simulink model "platoon_NRMPC"  (R2024b)
settings: Solver=FixedStepAuto  StartTime=0.0  StopTime=240  FixedStep=d_t  RelTol=1e-3
values from neighbouring files (symbols this model uses):
  A_i = [0 1;0 0]    [design_script.m]    (also in platoon_implementation_variables.mat = [0  1; 0  0])
  act_est = cell(1,N)    [design_script.m]    (also in platoon_implementation_variables.mat = )
  amp_n_u_f = 2e-2    (= 0.02)    [design_script.m]    (also in platoon_implementation_variables.mat)
  amp_n_u_s1 = 1e-2    (= 0.01)    [design_script.m]    (also in platoon_implementation_variables.mat)
  amp_n_u_s2 = 1e-2    (= 0.01)    [design_script.m]    (also in platoon_implementation_variables.mat)
  amp_n_x = 1e-2    (= 0.01)    [design_script.m]    (also in platoon_implementation_variables.mat)
  B_i = [0;1]    [design_script.m]    (also in platoon_implementation_variables.mat = [0 1])
  C = [1 0]    [design_script.m]    (also in platoon_implementation_variables.mat)
  car_len_prev = [0 5*ones(1,N-1)]    [design_script.m]    (also in platoon_implementation_variables.mat = [0 5 5 5 5 5 5 5 5 5])
  Ch = [1 h]    [design_script.m]    (also in platoon_implementation_variables.mat = [1 5])
  d_t = 0.1    [design_script.m]    (also in platoon_implementation_variables.mat)
  G_act_c = cell(1,N)    [design_script.m]    (also in platoon_implementation_variables.mat = )
  K_D_implem =     [NRF_implem.mat]    (also in platoon_implementation_variables.mat)
  m = dims(3)    [car_MPC_follower.m]    (also in car_MPC_leader.m = dims(2); platoon_implementation_variables.mat = 1)
  n = dims(2)    [car_MPC_follower.m]    (also in car_MPC_leader.m = dims(1); platoon_implementation_variables.mat = 3)
  n_w = zeros(1,N)    [design_script.m]    (also in platoon_implementation_variables.mat = [1 1 1 1 1 1 1 1 1 1])
  pos_ref = h*10    (= 50)    [design_script.m]    (also in platoon_implementation_variables.mat)
  U_lims = 10 * ones(1,N)    [design_script.m]    (also in platoon_implementation_variables.mat = [10 10 10 10 10 10 10 10 10 10])
  x0_c = [9.38914167955 12.3528095305 0 -60.4298352947 12.5503912552 0 -103.066925889 9.67248980493 0 -164.188527826 9.84551868802 0 ... (30 elements, 3x10)]    [init_scatter.mat]    (also in platoon_implementation_variables.mat)
undefined symbols (not defined in the file or in its folder): car_MPC_follower, car_MPC_leader, DiscIntNeverNeededParam
settings Model: Creator=Andrei

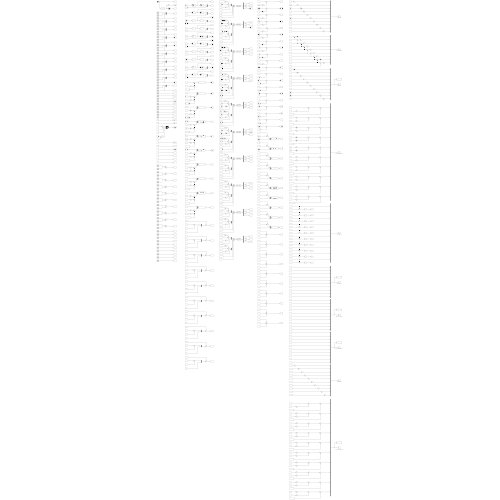
[thumbnail: Simulink's stored preview of the top-level diagram]
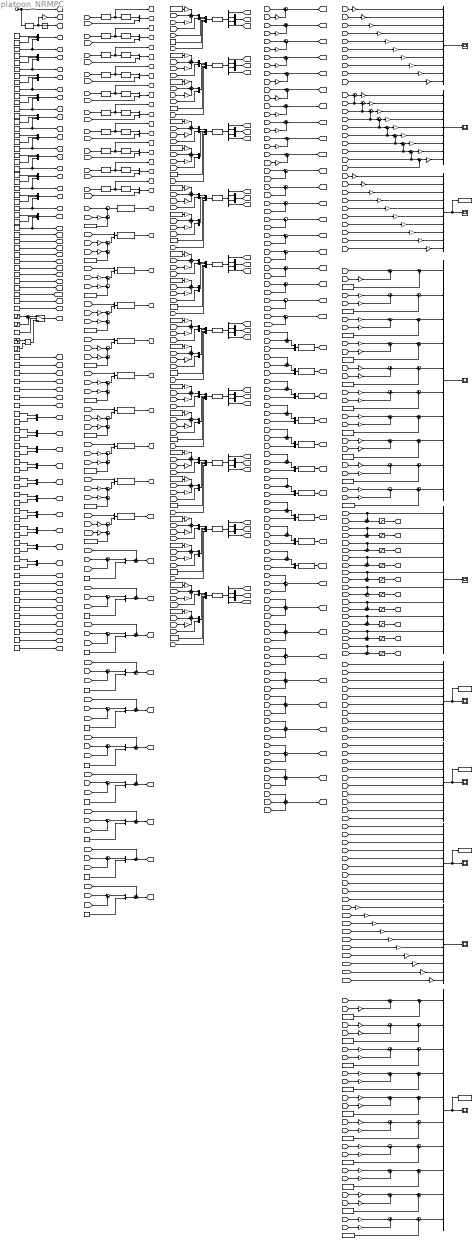
== system platoon_NRMPC ==
  " " : MATLABFcn  MATLABFcn=car_MPC_leader(u(1:n+n_w(1)),u(n+n_w(1)+1),u(n+n_w(1)+2:n+n_w(1)+3),u(n+n_w(1)+4))  OutputDimensions=n+m  SampleTime=d_t
  "  " : MATLABFcn  MATLABFcn=car_MPC_follower(u(1:n+n_w(2)),u(n+n_w(2)+1:2*n+n_w(1)+n_w(2)),u(2*n+n_w(1)+n_w(2)+1:2*n+n_w(1)+n_w(2)+3),u(2*n+n_w(1)+n_w(2)+4))  OutputDimensions=n+m  SampleTime=d_t
  "   " : MATLABFcn  MATLABFcn=car_MPC_follower(u(1:n+n_w(3)),u(n+n_w(3)+1:2*n+n_w(2)+n_w(3)),u(2*n+n_w(2)+n_w(3)+1:2*n+n_w(2)+n_w(3)+3),u(2*n+n_w(2)+n_w(3)+4))  OutputDimensions=n+m  SampleTime=d_t
  "    " : MATLABFcn  MATLABFcn=car_MPC_follower(u(1:n+n_w(4)),u(n+n_w(4)+1:2*n+n_w(3)+n_w(4)),u(2*n+n_w(3)+n_w(4)+1:2*n+n_w(3)+n_w(4)+3),u(2*n+n_w(3)+n_w(4)+4))  OutputDimensions=n+m  SampleTime=d_t
  "     " : MATLABFcn  MATLABFcn=car_MPC_follower(u(1:n+n_w(5)),u(n+n_w(5)+1:2*n+n_w(4)+n_w(5)),u(2*n+n_w(4)+n_w(5)+1:2*n+n_w(4)+n_w(5)+3),u(2*n+n_w(4)+n_w(5)+4))  OutputDimensions=n+m  SampleTime=d_t
  "      " : MATLABFcn  MATLABFcn=car_MPC_follower(u(1:n+n_w(6)),u(n+n_w(6)+1:2*n+n_w(5)+n_w(6)),u(2*n+n_w(5)+n_w(6)+1:2*n+n_w(5)+n_w(6)+3),u(2*n+n_w(5)+n_w(6)+4))  OutputDimensions=n+m  SampleTime=d_t
  "       " : MATLABFcn  MATLABFcn=car_MPC_follower(u(1:n+n_w(7)),u(n+n_w(7)+1:2*n+n_w(6)+n_w(7)),u(2*n+n_w(6)+n_w(7)+1:2*n+n_w(6)+n_w(7)+3),u(2*n+n_w(6)+n_w(7)+4))  OutputDimensions=n+m  SampleTime=d_t
  "        " : MATLABFcn  MATLABFcn=car_MPC_follower(u(1:n+n_w(8)),u(n+n_w(8)+1:2*n+n_w(7)+n_w(8)),u(2*n+n_w(7)+n_w(8)+1:2*n+n_w(7)+n_w(8)+3),u(2*n+n_w(7)+n_w(8)+4))  OutputDimensions=n+m  SampleTime=d_t
  "         " : MATLABFcn  MATLABFcn=car_MPC_follower(u(1:n+n_w(9)),u(n+n_w(9)+1:2*n+n_w(8)+n_w(9)),u(2*n+n_w(8)+n_w(9)+1:2*n+n_w(8)+n_w(9)+3),u(2*n+n_w(8)+n_w(9)+4))  OutputDimensions=n+m  SampleTime=d_t
  "          " : MATLABFcn  MATLABFcn=car_MPC_follower(u(1:n+n_w(10)),u(n+n_w(10)+1:2*n+n_w(9)+n_w(10)),u(2*n+n_w(9)+n_w(10)+1:2*n+n_w(9)+n_w(10)+3),u(2*n+n_w(9)+n_w(10)+4))  OutputDimensions=n+m  SampleTime=d_t
  Clock1 : Clock
  Constant1 : Constant
  Constant{5..6,8..10,18,22..25,51..59} (19 alike) : Constant  Value=0  SampleTime=d_t
  Constant{11,33,37,64,74} (5 alike) : Constant  Value=car_len_prev(5)  SampleTime=d_t
  Constant{12,36,40,65,75} (5 alike) : Constant  Value=car_len_prev(6)  SampleTime=d_t
  Constant{13,39,43,66,76} (5 alike) : Constant  Value=car_len_prev(7)  SampleTime=d_t
  Constant{14,42,46,67,77} (5 alike) : Constant  Value=car_len_prev(8)  SampleTime=d_t
  Constant{15,45,49,68,78} (5 alike) : Constant  Value=car_len_prev(9)  SampleTime=d_t
  Constant{16,48,69,79} (4 alike) : Constant  Value=car_len_prev(10)  SampleTime=d_t
  Constant{2,17,20,60,70} (5 alike) : Constant  Value=car_len_prev(1)  SampleTime=d_t
  Constant{4,19,28,61,71} (5 alike) : Constant  Value=car_len_prev(2)  SampleTime=d_t
  Constant21 : Constant  Value=[n; m]  SampleTime=d_t
  Constant26 : Constant  Value=[2; n; m]  SampleTime=d_t
  Constant{3,27,31,62,72} (5 alike) : Constant  Value=car_len_prev(3)  SampleTime=d_t
  Constant29 : Constant  Value=[3; n; m]  SampleTime=d_t
  Constant{7,30,34,63,73} (5 alike) : Constant  Value=car_len_prev(4)  SampleTime=d_t
  Constant32 : Constant  Value=[4; n; m]  SampleTime=d_t
  Constant35 : Constant  Value=[5; n; m]  SampleTime=d_t
  Constant38 : Constant  Value=[6; n; m]  SampleTime=d_t
  Constant41 : Constant  Value=[7; n; m]  SampleTime=d_t
  Constant44 : Constant  Value=[8; n; m]  SampleTime=d_t
  Constant47 : Constant  Value=[9; n; m]  SampleTime=d_t
  Constant50 : Constant  Value=[10; n; m]  SampleTime=d_t
  Demux{,1..9} (10 alike) : Demux
  Discrete State-Space : DiscreteStateSpace  A=K_D_implem{1}.a  B=K_D_implem{1}.b  C=K_D_implem{1}.c  D=K_D_implem{1}.d  SampleTime=d_t
  Discrete State-Space1 : DiscreteStateSpace  A=K_D_implem{2}.a  B=K_D_implem{2}.b  C=K_D_implem{2}.c  D=K_D_implem{2}.d  SampleTime=d_t
  Discrete State-Space10 : DiscreteStateSpace  A=act_est{1}.a  B=act_est{1}.b  C=act_est{1}.c  D=act_est{1}.d  SampleTime=d_t
  Discrete State-Space11 : DiscreteStateSpace  A=act_est{2}.a  B=act_est{2}.b  C=act_est{2}.c  D=act_est{2}.d  SampleTime=d_t
  Discrete State-Space12 : DiscreteStateSpace  A=act_est{3}.a  B=act_est{3}.b  C=act_est{3}.c  D=act_est{3}.d  SampleTime=d_t
  Discrete State-Space13 : DiscreteStateSpace  A=act_est{4}.a  B=act_est{4}.b  C=act_est{4}.c  D=act_est{4}.d  SampleTime=d_t
  Discrete State-Space14 : DiscreteStateSpace  A=act_est{5}.a  B=act_est{5}.b  C=act_est{5}.c  D=act_est{5}.d  SampleTime=d_t
  Discrete State-Space15 : DiscreteStateSpace  A=act_est{6}.a  B=act_est{6}.b  C=act_est{6}.c  D=act_est{6}.d  SampleTime=d_t
  Discrete State-Space16 : DiscreteStateSpace  A=act_est{7}.a  B=act_est{7}.b  C=act_est{7}.c  D=act_est{7}.d  SampleTime=d_t
  Discrete State-Space17 : DiscreteStateSpace  A=act_est{8}.a  B=act_est{8}.b  C=act_est{8}.c  D=act_est{8}.d  SampleTime=d_t
  Discrete State-Space18 : DiscreteStateSpace  A=act_est{9}.a  B=act_est{9}.b  C=act_est{9}.c  D=act_est{9}.d  SampleTime=d_t
  Discrete State-Space19 : DiscreteStateSpace  A=act_est{10}.a  B=act_est{10}.b  C=act_est{10}.c  D=act_est{10}.d  SampleTime=d_t
  Discrete State-Space2 : DiscreteStateSpace  A=K_D_implem{3}.a  B=K_D_implem{3}.b  C=K_D_implem{3}.c  D=K_D_implem{3}.d  SampleTime=d_t
  Discrete State-Space3 : DiscreteStateSpace  A=K_D_implem{4}.a  B=K_D_implem{4}.b  C=K_D_implem{4}.c  D=K_D_implem{4}.d  SampleTime=d_t
  Discrete State-Space4 : DiscreteStateSpace  A=K_D_implem{5}.a  B=K_D_implem{5}.b  C=K_D_implem{5}.c  D=K_D_implem{5}.d  SampleTime=d_t
  Discrete State-Space5 : DiscreteStateSpace  A=K_D_implem{6}.a  B=K_D_implem{6}.b  C=K_D_implem{6}.c  D=K_D_implem{6}.d  SampleTime=d_t
  Discrete State-Space6 : DiscreteStateSpace  A=K_D_implem{7}.a  B=K_D_implem{7}.b  C=K_D_implem{7}.c  D=K_D_implem{7}.d  SampleTime=d_t
  Discrete State-Space7 : DiscreteStateSpace  A=K_D_implem{8}.a  B=K_D_implem{8}.b  C=K_D_implem{8}.c  D=K_D_implem{8}.d  SampleTime=d_t
  Discrete State-Space8 : DiscreteStateSpace  A=K_D_implem{9}.a  B=K_D_implem{9}.b  C=K_D_implem{9}.c  D=K_D_implem{9}.d  SampleTime=d_t
  Discrete State-Space9 : DiscreteStateSpace  A=K_D_implem{10}.a  B=K_D_implem{10}.b  C=K_D_implem{10}.c  D=K_D_implem{10}.d  SampleTime=d_t
  Discrete-Time Integrator1 : DiscreteIntegrator  InitialCondition=pos_ref  SampleTime=d_t  ICPrevOutput=DiscIntNeverNeededParam  ICPrevScaledInput=DiscIntNeverNeededParam
  Fcn : Fcn  Expr=spd_ref*(u(1)>=0)+(3-spd_ref)*(u(1)>=40)+30*(u(1)>=120)-30*(u(1)>=130)
  Gain{1,3,29,56,58,60,62,64,66,68,139,142..143,145,147,149..150,152,154,157} (20 alike) : Gain  Gain=[Ch 0]  Multiplication=Matrix(K*u)
  Gain{2,4,6..16,18..28,38..39,42..55,57,59,61,63,65,67,71,141,144,146,148,151,153,155..156,158} (56 alike) : Gain  Gain=[C 0]  Multiplication=Matrix(K*u)
  Gain{69,76,78,80,82,84,86,88,90,92,94,96,98,100,102,104,106} (17 alike) : Gain  Gain=blkdiag(1,0,0)  Multiplication=Matrix(K*u)
  Gain{5,70,73..75,77,79,81,83,85,87,89,91,93,95,97,99,101,103,105,107} (21 alike) : Gain  Gain=[1;0;0]  Multiplication=Matrix(K*u)
  Gain108 : Gain  Gain=5  Multiplication=Matrix(K*u)
  Gain109 : Gain  Gain=6  Multiplication=Matrix(K*u)
  Gain110 : Gain  Gain=7  Multiplication=Matrix(K*u)
  Gain{111..120} (10 alike) : Gain  Gain=[0 1 0]  Multiplication=Matrix(K*u)
  Gain121 : Gain  Gain=8  Multiplication=Matrix(K*u)
  Gain122 : Gain  Gain=9  Multiplication=Matrix(K*u)
  Gain123 : Gain  Gain=10  Multiplication=Matrix(K*u)
  Gain124 : Gain  Multiplication=Matrix(K*u)
  Gain125 : Gain  Gain=2  Multiplication=Matrix(K*u)
  Gain126 : Gain  Gain=3  Multiplication=Matrix(K*u)
  Gain127 : Gain  Gain=4  Multiplication=Matrix(K*u)
  Gain17 : Gain  Gain=d_t
  Gain{30..37,40..41} (10 alike) : Gain  Gain=diag([1 1 0])  Multiplication=Matrix(K*u)
  MPC commands to NRF : Scope
  MPC commands to platoon : Scope
  MPC infeasibility : Scope
  Mux{,7..11,22..23,25,27} (10 alike) : Mux  Inputs=3
  Mux{1..6,15..19,21,24,26,28..46,48,50..52,54,56..57,59..61,63..65,67..69,71..73,75..77,79..81,83,85..103} (78 alike) : Mux  Inputs=2
  Mux{13..14,20,55,84,104..107} (9 alike) : Mux  Inputs=10
  Mux12 : Mux  Inputs=9
  Mux{47,49,53,58,62,66,70,74,78,82} (10 alike) : Mux
  NRF commands : Scope
  Product : Product
  Saturation : Saturate  UpperLimit=U_lims(1)  LowerLimit=-U_lims(1)
  Saturation1 : Saturate  UpperLimit=U_lims(2)  LowerLimit=-U_lims(2)
  Saturation2 : Saturate  UpperLimit=U_lims(3)  LowerLimit=-U_lims(3)
  Saturation3 : Saturate  UpperLimit=U_lims(4)  LowerLimit=-U_lims(4)
  Saturation4 : Saturate  UpperLimit=U_lims(5)  LowerLimit=-U_lims(5)
  Saturation5 : Saturate  UpperLimit=U_lims(6)  LowerLimit=-U_lims(6)
  Saturation6 : Saturate  UpperLimit=U_lims(7)  LowerLimit=-U_lims(7)
  Saturation7 : Saturate  UpperLimit=U_lims(8)  LowerLimit=-U_lims(8)
  Saturation8 : Saturate  UpperLimit=U_lims(9)  LowerLimit=-U_lims(9)
  Saturation9 : Saturate  UpperLimit=U_lims(10)  LowerLimit=-U_lims(10)
  Sine Wave : Sin  Amplitude=0.4*U_lims(3)  Frequency=0.2  Phase=pi  SampleTime=d_t
  State-Space : StateSpace  A=A_i  B=B_i  C=eye(2)  D=zeros(2,1)  InitialCondition=x0_c(1:2,1)
  State-Space1 : StateSpace  A=G_act_c{1}.a  B=G_act_c{1}.b  C=G_act_c{1}.c  D=G_act_c{1}.d  InitialCondition=x0_c(3,1)
  State-Space10 : StateSpace  A=A_i  B=B_i  C=eye(2)  D=zeros(2,1)  InitialCondition=x0_c(1:2,6)
  State-Space11 : StateSpace  A=G_act_c{6}.a  B=G_act_c{6}.b  C=G_act_c{6}.c  D=G_act_c{6}.d  InitialCondition=x0_c(3,6)
  State-Space12 : StateSpace  A=A_i  B=B_i  C=eye(2)  D=zeros(2,1)  InitialCondition=x0_c(1:2,10)
  State-Space13 : StateSpace  A=G_act_c{10}.a  B=G_act_c{10}.b  C=G_act_c{10}.c  D=G_act_c{10}.d  InitialCondition=x0_c(3,10)
  State-Space14 : StateSpace  A=A_i  B=B_i  C=eye(2)  D=zeros(2,1)  InitialCondition=x0_c(1:2,7)
  State-Space15 : StateSpace  A=G_act_c{7}.a  B=G_act_c{7}.b  C=G_act_c{7}.c  D=G_act_c{7}.d  InitialCondition=x0_c(3,7)
  State-Space16 : StateSpace  A=A_i  B=B_i  C=eye(2)  D=zeros(2,1)  InitialCondition=x0_c(1:2,8)
  State-Space17 : StateSpace  A=G_act_c{8}.a  B=G_act_c{8}.b  C=G_act_c{8}.c  D=G_act_c{8}.d  InitialCondition=x0_c(3,8)
  State-Space18 : StateSpace  A=A_i  B=B_i  C=eye(2)  D=zeros(2,1)  InitialCondition=x0_c(1:2,9)
  State-Space19 : StateSpace  A=G_act_c{9}.a  B=G_act_c{9}.b  C=G_act_c{9}.c  D=G_act_c{9}.d  InitialCondition=x0_c(3,9)
  State-Space2 : StateSpace  A=A_i  B=B_i  C=eye(2)  D=zeros(2,1)  InitialCondition=x0_c(1:2,2)
  State-Space3 : StateSpace  A=G_act_c{2}.a  B=G_act_c{2}.b  C=G_act_c{2}.c  D=G_act_c{2}.d  InitialCondition=x0_c(3,2)
  State-Space4 : StateSpace  A=A_i  B=B_i  C=eye(2)  D=zeros(2,1)  InitialCondition=x0_c(1:2,3)
  State-Space5 : StateSpace  A=G_act_c{3}.a  B=G_act_c{3}.b  C=G_act_c{3}.c  D=G_act_c{3}.d  InitialCondition=x0_c(3,3)
  State-Space6 : StateSpace  A=A_i  B=B_i  C=eye(2)  D=zeros(2,1)  InitialCondition=x0_c(1:2,4)
  State-Space7 : StateSpace  A=G_act_c{4}.a  B=G_act_c{4}.b  C=G_act_c{4}.c  D=G_act_c{4}.d  InitialCondition=x0_c(3,4)
  State-Space8 : StateSpace  A=A_i  B=B_i  C=eye(2)  D=zeros(2,1)  InitialCondition=x0_c(1:2,5)
  State-Space9 : StateSpace  A=G_act_c{5}.a  B=G_act_c{5}.b  C=G_act_c{5}.c  D=G_act_c{5}.d  InitialCondition=x0_c(3,5)
  Step : Step  Time=40  After=-2*U_lims(3)  SampleTime=d_t
  Step1 : Step  Time=40  After=2*U_lims(3)  SampleTime=d_t
  Step2 : Step  Time=40  SampleTime=d_t
  Sum{,1..2,4..5,8,11,13..14,22,28,30,32,34,36,38,40..44,46,48,53..54,99,109,111,113,115,117,119,121,123,125,127,129,132..133,135,138,140..141,144..145,147,150..152,155..156} (51 alike) : Sum  Inputs=|++
  Sum{3,7,10,52,55,130..131,134,136..137,139,142..143,146,148..149,153..154,157..158} (20 alike) : Sum  Inputs=|-+
  Sum{81,100..108} (10 alike) : Sum  Inputs=+++
  Sum{29,31,33,35,37,39,45,47,49..51,60..78,110,112,114,116,118,120,122,124,126,128} (40 alike) : Sum  Inputs=++|
  Sum{6,9,12,15..21,23..27,56..59} (19 alike) : Sum  Inputs=|+-
  Sum{79..80,82..98} (19 alike) : Sum  Inputs=++-
  Switch : Switch  Criteria=u2 > Threshold  SaturateOnIntegerOverflow=off  InputSameDT=off
  To Workspace : ToWorkspace  VariableName=y  SaveFormat=Timeseries  SampleTime=d_t
  To Workspace1 : ToWorkspace  VariableName=u_s2  SaveFormat=Timeseries  SampleTime=d_t
  To Workspace2 : ToWorkspace  VariableName=u_s1  SaveFormat=Timeseries  SampleTime=d_t
  To Workspace3 : ToWorkspace  VariableName=u_f  SaveFormat=Timeseries  SampleTime=d_t
  To Workspace4 : ToWorkspace  VariableName=v  SaveFormat=Timeseries  SampleTime=d_t
  Uniform Random Number{,1..17,28..39} (30 alike) : UniformRandomNumber  Minimum=-amp_n_x  Maximum=amp_n_x  Seed=randi(1e3)  SampleTime=d_t
  Uniform Random Number{18..27} (10 alike) : UniformRandomNumber  Minimum=-amp_n_u_f  Maximum=amp_n_u_f  Seed=randi(1e3)  SampleTime=d_t
  Uniform Random Number{40..59} (20 alike) : UniformRandomNumber  Minimum=-amp_n_u_s1  Maximum=amp_n_u_s1  Seed=randi(1e3)  SampleTime=d_t
  Uniform Random Number{60..69} (10 alike) : UniformRandomNumber  Minimum=-amp_n_u_s2  Maximum=amp_n_u_s2  Seed=randi(1e3)  SampleTime=d_t
  headway_based_distances : Scope
  intervehicle_distance : Scope
  length_based_interdistances : Scope
  total_commands : Scope
  vehicle position : Scope
  vehicle speed : Scope
  wires:
  Mux12/1 -> intervehicle_distance/1
  Sum29/1 -> Saturation/1
  Sum31/1 -> Saturation1/1
  Sum35/1 -> Saturation3/1
  Sum39/1 -> Saturation5/1
  Sum37/1 -> Saturation4/1
  [d_1] -> Sum29/2
  [d_2] -> Sum31/2
  [d_3] -> Sum33/2
  [d_4] -> Sum35/2
  [d_5] -> Sum37/2
  [d_6] -> Sum39/2
  [x_6] -> Gain11/1
  [x_1] -> Gain6/1
  [x_5] -> Gain10/1
  [x_4] -> Gain9/1
  [x_3] -> Gain8/1
  [x_2] -> Gain7/1
  Mux14/1 -> vehicle position/1
  Gain6/1 -> Mux14/1
  Gain7/1 -> Mux14/2
  Gain8/1 -> Mux14/3
  Gain9/1 -> Mux14/4
  Gain10/1 -> Mux14/5
  Gain11/1 -> Mux14/6
  Sum33/1 -> Saturation2/1
  Uniform Random Number21/1 -> [n_u_f_4]
  Uniform Random Number19/1 -> [n_u_f_2]
  Constant8/1 -> [d_4]
  Constant9/1 -> [d_5]
  Constant6/1 -> [d_2]
  Constant5/1 -> [d_1]
  Uniform Random Number22/1 -> [n_u_f_5]
  Sum/1 -> Switch/1
  Uniform Random Number18/1 -> [n_u_f_1]
  Uniform Random Number23/1 -> [n_u_f_6]
  Step/1 -> Sum/1
  Constant10/1 -> [d_6]
  Step1/1 -> Sum/2
  Uniform Random Number20/1 -> [n_u_f_3]
  Saturation/1 -> [u_1]
  Saturation1/1 -> [u_2]
  Saturation2/1 -> [u_3]
  Saturation3/1 -> [u_4]
  Saturation4/1 -> [u_5]
  Saturation5/1 -> [u_6]
  Sum14/1 -> [x_n_a_6]
  [x_2] -> Sum1/1
  Sum4/1 -> [x_n_a_1]
  [x_4] -> Sum8/1
  [n_x_1] -> Gain31/1
  [n_x_3] -> Gain32/1
  [x_6] -> Sum14/1
  [x_5] -> Sum11/1
  Sum8/1 -> [x_n_a_4]
  Gain31/1 -> Sum4/2
  Sum11/1 -> [x_n_a_5]
  Gain40/1 -> Sum11/2
  Gain41/1 -> Sum14/2
  Gain33/1 -> Sum8/2
  Gain30/1 -> Sum1/2
  [x_1] -> Sum4/1
  Gain32/1 -> Sum5/2
  [x_3] -> Sum5/1
  Sum5/1 -> [x_n_a_3]
  Sum1/1 -> [x_n_a_2]
  [n_x_2] -> Gain30/1
  [n_x_5] -> Gain40/1
  [n_x_4] -> Gain33/1
  [n_x_6] -> Gain41/1
  Mux24/1 -> [x_2]
  Mux30/1 -> [x_5]
  [u_5] -> State-Space9/1
  State-Space8/1 -> Mux30/1
  State-Space11/1 -> [a_6], State-Space10/1
  State-Space3/1 -> [a_2], State-Space2/1
  State-Space5/1 -> [a_3], State-Space4/1
  Mux28/1 -> [x_4]
  State-Space4/1 -> Mux26/1
  [u_2] -> State-Space3/1
  Mux33/1 -> [x_1]
  [u_1] -> State-Space1/1
  Mux26/1 -> [x_3]
  State-Space1/1 -> [a_1], State-Space/1
  Mux32/1 -> [x_6]
  State-Space7/1 -> [a_4], State-Space6/1
  [u_4] -> State-Space7/1
  [u_6] -> State-Space11/1
  State-Space6/1 -> Mux28/1
  State-Space2/1 -> Mux24/1
  [u_3] -> State-Space5/1
  State-Space10/1 -> Mux32/1
  State-Space/1 -> Mux33/1
  State-Space9/1 -> [a_5], State-Space8/1
  Constant22/1 -> [d_9]
  Constant24/1 -> [d_8]
  Constant23/1 -> [d_7]
  Constant25/1 -> [d_10]
  Uniform Random Number25/1 -> [n_u_f_8]
  Uniform Random Number24/1 -> [n_u_f_7]
  Uniform Random Number26/1 -> [n_u_f_9]
  Gain36/1 -> Sum40/2
  Gain35/1 -> Sum43/2
  Sum41/1 -> [x_n_a_10]
  Sum43/1 -> [x_n_a_8]
  [n_x_7] -> Gain34/1
  Gain34/1 -> Sum42/2
  Gain37/1 -> Sum41/2
  [x_8] -> Sum43/1
  Sum40/1 -> [x_n_a_9]
  Sum42/1 -> [x_n_a_7]
  [n_x_9] -> Gain36/1
  [n_x_8] -> Gain35/1
  [x_10] -> Sum41/1
  [x_9] -> Sum40/1
  [x_7] -> Sum42/1
  [n_x_10] -> Gain37/1
  Sum47/1 -> Saturation7/1
  [d_9] -> Sum49/2
  Sum49/1 -> Saturation8/1
  Saturation7/1 -> [u_8]
  Saturation6/1 -> [u_7]
  Saturation9/1 -> [u_10]
  Sum51/1 -> Saturation9/1
  [d_10] -> Sum51/2
  [d_7] -> Sum45/2
  Saturation8/1 -> [u_9]
  [d_8] -> Sum47/2
  Sum45/1 -> Saturation6/1
  Mux20/1 -> total_commands/1
  Gain12/1 -> Mux12/1
  Gain13/1 -> Mux12/2
  Gain14/1 -> Mux12/3
  Gain15/1 -> Mux12/4
  Gain16/1 -> Mux12/5
  Gain48/1 -> Mux12/6
  Gain49/1 -> Mux12/7
  Gain50/1 -> Mux12/8
  Gain51/1 -> Mux12/9
  [x_1] -> Sum19/1
  Sum19/1 -> Gain12/1
  [x_2] -> Sum19/2, Sum17/1
  Sum17/1 -> Gain13/1
  Sum18/1 -> Gain14/1
  Sum20/1 -> Gain15/1
  Sum21/1 -> Gain16/1
  Sum56/1 -> Gain48/1
  Sum57/1 -> Gain49/1
  Sum58/1 -> Gain50/1
  Sum59/1 -> Gain51/1
  [x_3] -> Sum17/2, Sum18/1
  [x_4] -> Sum18/2, Sum20/1
  [x_5] -> Sum20/2, Sum21/1
  [x_6] -> Sum21/2, Sum56/1
  [x_7] -> Sum56/2, Sum57/1
  [x_8] -> Sum57/2, Sum58/1
  [x_9] -> Sum58/2, Sum59/1
  [x_10] -> Sum59/2
  [x_7] -> Gain52/1
  Gain52/1 -> Mux14/7
  [x_8] -> Gain53/1
  Gain53/1 -> Mux14/8
  [x_9] -> Gain54/1
  Gain54/1 -> Mux14/9
  [x_10] -> Gain55/1
  Gain55/1 -> Mux14/10
  State-Space19/1 -> [a_9], State-Space18/1
  Mux40/1 -> [x_10]
  Mux39/1 -> [x_9]
  [u_10] -> State-Space13/1
  [u_7] -> State-Space15/1
  State-Space12/1 -> Mux40/1
  State-Space16/1 -> Mux38/1
  State-Space17/1 -> [a_8], State-Space16/1
  State-Space13/1 -> [a_10], State-Space12/1
  Mux38/1 -> [x_8]
  State-Space14/1 -> Mux37/1
  Mux37/1 -> [x_7]
  [u_8] -> State-Space17/1
  State-Space18/1 -> Mux39/1
  [u_9] -> State-Space19/1
  State-Space15/1 -> [a_7], State-Space14/1
  [u_c_1] -> Sum29/1, Mux20/1
  [u_c_2] -> Sum31/1, Mux20/2
  [u_c_3] -> Sum33/1, Mux20/3
  [u_c_4] -> Sum35/1, Mux20/4
  [u_c_6] -> Sum39/1, Mux20/6
  [u_c_5] -> Sum37/1, Mux20/5
  [u_c_8] -> Sum47/1, Mux20/8
  [u_c_7] -> Sum45/1, Mux20/7
  [u_c_9] -> Sum49/1, Mux20/9
  [u_c_10] -> Sum51/1, Mux20/10
  [u_f_2_n] -> Mux2/1
  [u_f_3_n] -> Mux3/1
  Sum12/1 -> Mux2/2
  [f_1] -> Gain1/1
  Gain56/1 -> Sum73/1
  Mux3/1 -> Discrete State-Space3/1
  Gain59/1 -> Sum12/1
  Sum23/1 -> Mux6/2
  [x_n_a_3] -> Gain28/1
  Mux4/1 -> Discrete State-Space4/1
  Gain4/1 -> Sum16/1
  Gain57/1 -> Sum23/1
  [f_6] -> Gain58/1
  [x_n_a_5] -> Gain57/1
  Sum16/1 -> Mux4/2
  [x_n_a_4] -> Gain4/1
  Gain28/1 -> Sum15/1
  [f_4] -> Gain29/1
  Gain29/1 -> Sum72/1
  [u_f_4_n] -> Mux4/1
  [f_5] -> Gain56/1
  [x_n_a_2] -> Gain59/1
  Gain58/1 -> Sum74/1
  Gain3/1 -> Sum70/1
  Sum15/1 -> Mux3/2
  [f_3] -> Gain60/1
  Mux2/1 -> Discrete State-Space2/1
  Sum9/1 -> Mux1/2
  Gain60/1 -> Sum71/1
  [u_f_1_n] -> Mux1/1
  Mux1/1 -> Discrete State-Space1/1
  Gain2/1 -> Sum9/1
  [f_2] -> Gain3/1
  [r] -> Sum6/1
  [x_n_a_1] -> Gain2/1
  Sum6/1 -> Discrete State-Space/1
  Gain1/1 -> Sum69/1
  [u_f_5_n] -> Mux6/1
  Mux6/1 -> Discrete State-Space5/1
  [u_f_9_n] -> Mux17/1
  Gain68/1 -> Sum75/1
  Mux5/1 -> Discrete State-Space6/1
  [f_9] -> Gain64/1
  [f_7] -> Gain68/1
  Gain66/1 -> Sum78/1
  Sum25/1 -> Mux15/2
  [f_8] -> Gain62/1
  Gain61/1 -> Sum25/1
  [u_f_8_n] -> Mux16/1
  Gain62/1 -> Sum76/1
  Sum26/1 -> Mux16/2
  [x_n_a_9] -> Gain65/1
  Mux16/1 -> Discrete State-Space8/1
  Gain63/1 -> Sum26/1
  [x_n_a_8] -> Gain63/1
  [x_n_a_6] -> Gain67/1
  [x_n_a_7] -> Gain61/1
  Gain67/1 -> Sum24/1
  [u_f_6_n] -> Mux5/1
  [u_f_7_n] -> Mux15/1
  Gain65/1 -> Sum27/1
  Mux17/1 -> Discrete State-Space9/1
  Gain64/1 -> Sum77/1
  Sum27/1 -> Mux17/2
  [f_10] -> Gain66/1
  Sum24/1 -> Mux5/2
  Mux15/1 -> Discrete State-Space7/1
  Sum28/1 -> [u_f_1_n]
  [n_u_f_1] -> Sum28/2
  [u_f_1] -> Sum28/1
  [u_f_2] -> Sum30/1
  Sum30/1 -> [u_f_2_n]
  [n_u_f_2] -> Sum30/2
  [u_f_3] -> Sum32/1
  Sum32/1 -> [u_f_3_n]
  [n_u_f_3] -> Sum32/2
  [n_u_f_6] -> Sum38/2
  [u_f_4] -> Sum34/1
  [u_f_6] -> Sum38/1
  Sum34/1 -> [u_f_4_n]
  [u_f_5] -> Sum36/1
  Sum38/1 -> [u_f_6_n]
  [n_u_f_5] -> Sum36/2
  Sum36/1 -> [u_f_5_n]
  [n_u_f_4] -> Sum34/2
  [n_u_f_9] -> Sum48/2
  [u_f_7] -> Sum44/1
  [u_f_9] -> Sum48/1
  Sum44/1 -> [u_f_7_n]
  [u_f_8] -> Sum46/1
  Sum48/1 -> [u_f_9_n]
  [n_u_f_8] -> Sum46/2
  Sum46/1 -> [u_f_8_n]
  [n_u_f_7] -> Sum44/2
  Sine Wave/1 -> Product/1
  Step2/1 -> Product/2
  Switch/1 -> [d_3]
  Constant1/1 -> Switch/2
  Product/1 -> Switch/3
  [u_9] -> Mux41/2
  [n_a_8] -> Sum64/2
  Sum65/1 -> Mux41/1
  Sum60/1 -> Mux29/1
  [u_4] -> Mux29/2
  [a_4] -> Sum60/1
  [n_a_5] -> Sum61/2
  [a_6] -> Sum62/1
  [u_6] -> Mux36/2
  [u_5] -> Mux31/2
  Discrete State-Space12/1 -> [act_x_3]
  [n_a_1] -> Sum67/2
  Discrete State-Space14/1 -> [act_x_5]
  [u_3] -> Mux21/2
  Mux35/1 -> Discrete State-Space17/1
  Discrete State-Space10/1 -> [act_x_1]
  Mux31/1 -> Discrete State-Space14/1
  Sum50/1 -> Mux21/1
  Discrete State-Space17/1 -> [act_x_8]
  Sum63/1 -> Mux34/1
  [u_2] -> Mux19/2
  [a_2] -> Sum68/1
  Mux42/1 -> Discrete State-Space19/1
  [a_1] -> Sum67/1
  [a_10] -> Sum66/1
  Sum61/1 -> Mux31/1
  Discrete State-Space18/1 -> [act_x_9]
  Discrete State-Space19/1 -> [act_x_10]
  [n_a_10] -> Sum66/2
  Mux21/1 -> Discrete State-Space12/1
  Sum68/1 -> Mux19/1
  Sum66/1 -> Mux42/1
  [a_3] -> Sum50/1
  [a_8] -> Sum64/1
  [u_1] -> Mux18/2
  Discrete State-Space11/1 -> [act_x_2]
  [n_a_7] -> Sum63/2
  Sum62/1 -> Mux36/1
  [u_8] -> Mux35/2
  [n_a_9] -> Sum65/2
  [n_a_6] -> Sum62/2
  [u_10] -> Mux42/2
  Mux18/1 -> Discrete State-Space10/1
  [a_7] -> Sum63/1
  Discrete State-Space13/1 -> [act_x_4]
  Mux41/1 -> Discrete State-Space18/1
  Sum64/1 -> Mux35/1
  Sum67/1 -> Mux18/1
  [a_9] -> Sum65/1
  Mux29/1 -> Discrete State-Space13/1
  [n_a_4] -> Sum60/2
  [a_5] -> Sum61/1
  [u_7] -> Mux34/2
  Discrete State-Space16/1 -> [act_x_7]
  [n_a_2] -> Sum68/2
  [n_a_3] -> Sum50/2
  Mux36/1 -> Discrete State-Space15/1
  Mux19/1 -> Discrete State-Space11/1
  Discrete State-Space15/1 -> [act_x_6]
  Mux34/1 -> Discrete State-Space16/1
  [act_x_1] -> Mux33/2
  [act_x_3] -> Mux26/2
  [act_x_2] -> Mux24/2
  [act_x_4] -> Mux28/2
  [act_x_5] -> Mux30/2
  [act_x_6] -> Mux32/2
  [act_x_7] -> Mux37/2
  [act_x_8] -> Mux38/2
  [act_x_9] -> Mux39/2
  [act_x_10] -> Mux40/2
  Discrete State-Space8/1 -> [u_f_9]
  Discrete State-Space/1 -> [u_f_1]
  Discrete State-Space1/1 -> [u_f_2]
  Discrete State-Space2/1 -> [u_f_3]
  Discrete State-Space3/1 -> [u_f_4]
  Discrete State-Space4/1 -> [u_f_5]
  Discrete State-Space5/1 -> [u_f_6]
  Discrete State-Space9/1 -> [u_f_10]
  Discrete State-Space7/1 -> [u_f_8]
  Discrete State-Space6/1 -> [u_f_7]
  Uniform Random Number/1 -> Mux/1
  Mux11/1 -> [n_x_6]
  Uniform Random Number34/1 -> Mux23/2
  Mux27/1 -> [n_x_8]
  Uniform Random Number30/1 -> Mux22/1
  Uniform Random Number31/1 -> Mux22/2
  Uniform Random Number37/1 -> Mux25/2
  Mux25/1 -> [n_x_7]
  Uniform Random Number28/1 -> Mux27/2
  Uniform Random Number8/1 -> [n_a_3], Mux8/3
  Uniform Random Number10/1 -> Mux9/2
  Uniform Random Number38/1 -> [n_a_7], Mux25/3
  Uniform Random Number1/1 -> Mux/2
  Uniform Random Number13/1 -> Mux10/2
  Uniform Random Number11/1 -> [n_a_4], Mux9/3
  Uniform Random Number35/1 -> [n_a_10], Mux23/3
  Uniform Random Number12/1 -> Mux10/1
  Uniform Random Number2/1 -> [n_a_1], Mux/3
  Uniform Random Number16/1 -> Mux11/2
  Uniform Random Number9/1 -> Mux9/1
  Mux8/1 -> [n_x_3]
  Uniform Random Number7/1 -> Mux8/2
  Uniform Random Number14/1 -> [n_a_5], Mux10/3
  Uniform Random Number17/1 -> [n_a_6], Mux11/3
  Mux22/1 -> [n_x_9]
  Uniform Random Number36/1 -> Mux25/1
  Mux/1 -> [n_x_1]
  Uniform Random Number39/1 -> Mux27/1
  Uniform Random Number15/1 -> Mux11/1
  Uniform Random Number29/1 -> [n_a_8], Mux27/3
  Mux7/1 -> [n_x_2]
  Uniform Random Number33/1 -> Mux23/1
  Mux10/1 -> [n_x_5]
  Uniform Random Number5/1 -> [n_a_2], Mux7/3
  Uniform Random Number32/1 -> [n_a_9], Mux22/3
  Uniform Random Number3/1 -> Mux7/1
  Mux9/1 -> [n_x_4]
  Uniform Random Number4/1 -> Mux7/2
  Mux23/1 -> [n_x_10]
  Uniform Random Number6/1 -> Mux8/1
  Constant2/1 -> Sum69/2
  Sum69/1 -> Sum6/2
  Constant4/1 -> Sum70/2
  Sum70/1 -> Sum9/2
  Constant3/1 -> Sum71/2
  Sum71/1 -> Sum12/2
  Constant7/1 -> Sum72/2
  Sum72/1 -> Sum15/2
  Constant11/1 -> Sum73/2
  Sum73/1 -> Sum16/2
  Constant12/1 -> Sum74/2
  Sum74/1 -> Sum23/2
  Constant13/1 -> Sum75/2
  Sum75/1 -> Sum24/2
  Constant14/1 -> Sum76/2
  Sum76/1 -> Sum25/2
  Constant15/1 -> Sum77/2
  Sum77/1 -> Sum26/2
  Constant16/1 -> Sum78/2
  Sum78/1 -> Sum27/2
  [u_f_4] -> Mux55/4
  [u_f_6] -> Mux55/6
  [u_f_1] -> Mux55/1
  [u_f_3] -> Mux55/3
  [u_f_10] -> Mux55/10
  [u_f_8] -> Mux55/8
  [u_f_7] -> Mux55/7
  [u_f_9] -> Mux55/9
  [u_f_5] -> Mux55/5
  [u_f_2] -> Mux55/2
  Mux55/1 -> To Workspace3/1, NRF commands/1
  Sum79/1 -> Mux44/1
  [u_f_1_n] -> Mux44/2
  Mux44/1 -> Mux47/1
  Mux47/1 -> " "/1
  " "/1 -> Demux/1
  Constant21/1 -> Mux47/3
  Demux/1 -> [u_s2_1]
  Demux/3 -> Mux48/2
  Demux/2 -> Mux48/1
  Mux48/1 -> [u_s1_1]
  Demux/4 -> [infeas_1]
  [r] -> Gain5/1
  Constant17/1 -> Gain70/1
  Gain5/1 -> Sum79/3
  [x_n_a_1] -> Sum79/2
  Gain70/1 -> Sum79/1
  Demux1/2 -> Mux50/1
  Gain73/1 -> Sum80/1
  Sum82/1 -> Mux45/1
  Demux1/1 -> [u_s2_2]
  Mux49/1 -> "  "/1
  Mux45/1 -> Mux49/2
  Constant26/1 -> Mux49/3
  Gain69/1 -> Sum80/3
  [x_n_a_1] -> Sum82/2
  Demux1/3 -> Mux50/2
  Mux46/1 -> Mux49/1
  [r] -> Gain74/1
  Gain75/1 -> Sum82/1
  Sum80/1 -> Mux46/1
  Mux50/1 -> [u_s1_2]
  Gain74/1 -> Sum82/3
  Constant19/1 -> Gain73/1
  "  "/1 -> Demux1/1
  [u_f_1_n] -> Mux45/2
  [u_f_2_n] -> Mux46/2
  Demux1/4 -> [infeas_2]
  [x_n_a_2] -> Sum80/2
  Constant20/1 -> Gain75/1
  [x_n_a_1] -> Gain69/1
  Constant27/1 -> Gain77/1
  Gain76/1 -> Sum83/3
  [u_f_2_n] -> Mux51/2
  Mux52/1 -> Mux53/1
  Mux53/1 -> "   "/1
  Gain77/1 -> Sum83/1
  Mux51/1 -> Mux53/2
  Constant28/1 -> Gain79/1
  Mux54/1 -> [u_s1_3]
  Sum83/1 -> Mux52/1
  Demux2/3 -> Mux54/2
  [u_f_3_n] -> Mux52/2
  [x_n_a_2] -> Gain76/1
  Sum84/1 -> Mux51/1
  Gain78/1 -> Sum84/3
  [x_n_a_3] -> Sum83/2
  Demux2/4 -> [infeas_3]
  [x_n_a_2] -> Sum84/2
  Constant29/1 -> Mux53/3
  Gain79/1 -> Sum84/1
  Demux2/1 -> [u_s2_3]
  Demux2/2 -> Mux54/1
  "   "/1 -> Demux2/1
  Mux56/1 -> Mux58/2
  [x_n_a_4] -> Sum85/2
  Sum86/1 -> Mux56/1
  Gain83/1 -> Sum86/1
  Constant32/1 -> Mux58/3
  "    "/1 -> Demux3/1
  Gain82/1 -> Sum86/3
  [u_f_4_n] -> Mux57/2
  Gain80/1 -> Sum85/3
  Constant31/1 -> Gain83/1
  Constant30/1 -> Gain81/1
  [u_f_3_n] -> Mux56/2
  [x_n_a_3] -> Sum86/2
  Sum85/1 -> Mux57/1
  Gain81/1 -> Sum85/1
  Demux3/4 -> [infeas_4]
  Mux59/1 -> [u_s1_4]
  Mux58/1 -> "    "/1
  [x_n_a_2] -> Gain82/1
  Demux3/1 -> [u_s2_4]
  Demux3/3 -> Mux59/2
  Demux3/2 -> Mux59/1
  [x_n_a_3] -> Gain80/1
  Mux57/1 -> Mux58/1
  [x_n_a_1] -> Gain78/1
  Sum87/1 -> Mux61/1
  [x_n_a_4] -> Gain84/1
  Demux4/4 -> [infeas_5]
  Gain86/1 -> Sum88/3
  Gain84/1 -> Sum87/3
  Demux4/1 -> [u_s2_5]
  Gain87/1 -> Sum88/1
  [x_n_a_4] -> Sum88/2
  Mux63/1 -> [u_s1_5]
  Mux60/1 -> Mux62/2
  [x_n_a_5] -> Sum87/2
  Constant35/1 -> Mux62/3
  Constant33/1 -> Gain85/1
  Gain85/1 -> Sum87/1
  Demux4/2 -> Mux63/1
  "     "/1 -> Demux4/1
  Demux4/3 -> Mux63/2
  [u_f_5_n] -> Mux61/2
  Constant34/1 -> Gain87/1
  Sum88/1 -> Mux60/1
  [x_n_a_3] -> Gain86/1
  Mux62/1 -> "     "/1
  Mux61/1 -> Mux62/1
  [u_f_4_n] -> Mux60/2
  Mux64/1 -> Mux66/2
  Demux5/4 -> [infeas_6]
  Gain88/1 -> Sum89/3
  Gain91/1 -> Sum90/1
  [u_f_6_n] -> Mux65/2
  Demux5/3 -> Mux67/2
  [x_n_a_5] -> Sum90/2
  [x_n_a_4] -> Gain90/1
  Mux65/1 -> Mux66/1
  Mux67/1 -> [u_s1_6]
  Demux5/2 -> Mux67/1
  Gain90/1 -> Sum90/3
  "      "/1 -> Demux5/1
  Sum89/1 -> Mux65/1
  [x_n_a_5] -> Gain88/1
  [x_n_a_6] -> Sum89/2
  [u_f_5_n] -> Mux64/2
  Constant38/1 -> Mux66/3
  Constant37/1 -> Gain91/1
  Demux5/1 -> [u_s2_6]
  Sum90/1 -> Mux64/1
  Gain89/1 -> Sum89/1
  Mux66/1 -> "      "/1
  Constant36/1 -> Gain89/1
  "       "/1 -> Demux6/1
  Gain94/1 -> Sum92/3
  [u_f_7_n] -> Mux69/2
  Gain93/1 -> Sum91/1
  Sum91/1 -> Mux69/1
  Mux70/1 -> "       "/1
  Gain95/1 -> Sum92/1
  Constant39/1 -> Gain93/1
  Demux6/4 -> [infeas_7]
  Demux6/2 -> Mux71/1
  Mux68/1 -> Mux70/2
  [x_n_a_6] -> Gain92/1
  Demux6/3 -> Mux71/2
  Demux6/1 -> [u_s2_7]
  Constant40/1 -> Gain95/1
  [u_f_6_n] -> Mux68/2
  [x_n_a_7] -> Sum91/2
  [x_n_a_5] -> Gain94/1
  [x_n_a_6] -> Sum92/2
  Gain92/1 -> Sum91/3
  Sum92/1 -> Mux68/1
  Mux69/1 -> Mux70/1
  Constant41/1 -> Mux70/3
  Mux71/1 -> [u_s1_7]
  [x_n_a_6] -> Gain98/1
  Demux7/4 -> [infeas_8]
  [x_n_a_8] -> Sum93/2
  Mux74/1 -> "        "/1
  Gain96/1 -> Sum93/3
  Gain98/1 -> Sum94/3
  [u_f_7_n] -> Mux72/2
  Demux7/1 -> [u_s2_8]
  [x_n_a_7] -> Sum94/2
  Constant42/1 -> Gain97/1
  Sum94/1 -> Mux72/1
  Mux75/1 -> [u_s1_8]
  Gain99/1 -> Sum94/1
  Sum93/1 -> Mux73/1
  Constant43/1 -> Gain99/1
  Gain97/1 -> Sum93/1
  [u_f_8_n] -> Mux73/2
  Mux73/1 -> Mux74/1
  "        "/1 -> Demux7/1
  Demux7/2 -> Mux75/1
  Demux7/3 -> Mux75/2
  Mux72/1 -> Mux74/2
  Constant44/1 -> Mux74/3
  [x_n_a_7] -> Gain96/1
  Constant45/1 -> Gain101/1
  Sum95/1 -> Mux77/1
  Mux76/1 -> Mux78/2
  Gain102/1 -> Sum96/3
  Demux8/1 -> [u_s2_9]
  [x_n_a_9] -> Sum95/2
  Sum96/1 -> Mux76/1
  [x_n_a_7] -> Gain102/1
  Demux8/3 -> Mux79/2
  "         "/1 -> Demux8/1
  Demux8/4 -> [infeas_9]
  Constant46/1 -> Gain103/1
  [x_n_a_8] -> Gain100/1
  Gain100/1 -> Sum95/3
  [u_f_8_n] -> Mux76/2
  Gain103/1 -> Sum96/1
  Mux77/1 -> Mux78/1
  Constant47/1 -> Mux78/3
  [x_n_a_8] -> Sum96/2
  [u_f_9_n] -> Mux77/2
  Demux8/2 -> Mux79/1
  Mux78/1 -> "         "/1
  Mux79/1 -> [u_s1_9]
  Gain101/1 -> Sum95/1
  [x_n_a_9] -> Gain104/1
  [x_n_a_8] -> Gain106/1
  Gain104/1 -> Sum97/3
  [x_n_a_9] -> Sum98/2
  Mux81/1 -> Mux82/1
  Sum98/1 -> Mux80/1
  Demux9/2 -> Mux83/1
  Constant48/1 -> Gain105/1
  Gain105/1 -> Sum97/1
  Mux83/1 -> [u_s1_10]
  Mux80/1 -> Mux82/2
  "          "/1 -> Demux9/1
  [u_f_9_n] -> Mux80/2
  Constant49/1 -> Gain107/1
  Sum97/1 -> Mux81/1
  Gain107/1 -> Sum98/1
  Demux9/1 -> [u_s2_10]
  [x_n_a_10] -> Sum97/2
  [u_f_10_n] -> Mux81/2
  Mux82/1 -> "          "/1
  Demux9/4 -> [infeas_10]
  Gain106/1 -> Sum98/3
  Demux9/3 -> Mux83/2
  Constant50/1 -> Mux82/3
  [u_f_10] -> Sum99/1
  [n_u_f_10] -> Sum99/2
  Sum99/1 -> [u_f_10_n]
  Uniform Random Number27/1 -> [n_u_f_10]
  [infeas_8] -> Gain121/1
  [infeas_1] -> Gain124/1
  Gain127/1 -> Mux84/4
  [infeas_2] -> Gain125/1
  Gain126/1 -> Mux84/3
  [infeas_3] -> Gain126/1
  [infeas_7] -> Gain110/1
  [infeas_5] -> Gain108/1
  Gain121/1 -> Mux84/8
  Gain123/1 -> Mux84/10
  [infeas_4] -> Gain127/1
  Gain109/1 -> Mux84/6
  [infeas_10] -> Gain123/1
  Gain108/1 -> Mux84/5
  Gain125/1 -> Mux84/2
  [infeas_6] -> Gain109/1
  Gain110/1 -> Mux84/7
  [infeas_9] -> Gain122/1
  Gain122/1 -> Mux84/9
  Gain124/1 -> Mux84/1
  Mux84/1 -> MPC infeasibility/1
  Uniform Random Number40/1 -> Mux85/1
  Uniform Random Number41/1 -> Mux85/2
  Mux85/1 -> [n_s1_1]
  Uniform Random Number43/1 -> Mux86/2
  Uniform Random Number42/1 -> Mux86/1
  Mux86/1 -> [n_s1_2]
  Uniform Random Number46/1 -> Mux88/1
  Uniform Random Number44/1 -> Mux87/1
  Uniform Random Number45/1 -> Mux87/2
  Mux88/1 -> [n_s1_4]
  Uniform Random Number47/1 -> Mux88/2
  Mux87/1 -> [n_s1_3]
  Uniform Random Number50/1 -> Mux90/1
  Uniform Random Number48/1 -> Mux89/1
  Uniform Random Number49/1 -> Mux89/2
  Mux90/1 -> [n_s1_6]
  Uniform Random Number53/1 -> Mux91/2
  Uniform Random Number55/1 -> Mux92/2
  Uniform Random Number54/1 -> Mux92/1
  Uniform Random Number51/1 -> Mux90/2
  Mux91/1 -> [n_s1_7]
  Mux92/1 -> [n_s1_8]
  Uniform Random Number52/1 -> Mux91/1
  Mux89/1 -> [n_s1_5]
  Uniform Random Number56/1 -> Mux93/1
  Mux94/1 -> [n_s1_10]
  Uniform Random Number57/1 -> Mux93/2
  Uniform Random Number59/1 -> Mux94/2
  Mux93/1 -> [n_s1_9]
  Uniform Random Number58/1 -> Mux94/1
  Uniform Random Number60/1 -> [n_s2_1]
  Uniform Random Number61/1 -> [n_s2_2]
  Uniform Random Number63/1 -> [n_s2_4]
  Uniform Random Number62/1 -> [n_s2_3]
  Uniform Random Number67/1 -> [n_s2_8]
  Uniform Random Number66/1 -> [n_s2_7]
  Uniform Random Number64/1 -> [n_s2_5]
  Uniform Random Number65/1 -> [n_s2_6]
  Uniform Random Number68/1 -> [n_s2_9]
  Uniform Random Number69/1 -> [n_s2_10]
  [d_r] -> Mux47/2
  Sum81/1 -> [u_c_1]
  [u_f_1] -> Sum81/1
  [u_s2_1] -> Sum81/2
  [n_s2_1] -> Sum81/3
  Sum100/1 -> [u_c_2]
  [u_s2_2] -> Sum100/2
  [u_f_2] -> Sum100/1
  [n_s2_2] -> Sum100/3
  Sum102/1 -> [u_c_3]
  [u_s2_3] -> Sum102/2
  [n_s2_4] -> Sum101/3
  [n_s2_3] -> Sum102/3
  Sum101/1 -> [u_c_4]
  [u_f_3] -> Sum102/1
  [u_f_4] -> Sum101/1
  [u_s2_4] -> Sum101/2
  [u_s2_7] -> Sum105/2
  [u_s2_8] -> Sum104/2
  Sum106/1 -> [u_c_5]
  [n_s2_7] -> Sum105/3
  Sum104/1 -> [u_c_8]
  [u_f_7] -> Sum105/1
  [u_s2_5] -> Sum106/2
  [u_f_6] -> Sum103/1
  [u_f_8] -> Sum104/1
  [u_f_5] -> Sum106/1
  [n_s2_5] -> Sum106/3
  [n_s2_6] -> Sum103/3
  Sum105/1 -> [u_c_7]
  [n_s2_8] -> Sum104/3
  [u_s2_6] -> Sum103/2
  Sum103/1 -> [u_c_6]
  Sum108/1 -> [u_c_9]
  [u_s2_10] -> Sum107/2
  [u_s2_9] -> Sum108/2
  [n_s2_9] -> Sum108/3
  [u_f_9] -> Sum108/1
  [u_f_10] -> Sum107/1
  [n_s2_10] -> Sum107/3
  Sum107/1 -> [u_c_10]
  [u_s1_1] -> Sum109/1
  [n_s1_1] -> Sum109/2
  [x_n_a_1] -> Sum110/1
  Mux43/1 -> Sum110/2
  Sum109/1 -> Mux43/1
  Constant18/1 -> Mux43/2
  Sum110/1 -> [f_1]
  Sum112/1 -> [f_2]
  [n_s1_2] -> Sum111/2
  [x_n_a_2] -> Sum112/1
  Sum111/1 -> Mux95/1
  [u_s1_2] -> Sum111/1
  Mux95/1 -> Sum112/2
  Constant51/1 -> Mux95/2
  Sum115/1 -> Mux97/1
  Constant52/1 -> Mux96/2
  Sum116/1 -> [f_4]
  [u_s1_4] -> Sum115/1
  [u_s1_3] -> Sum113/1
  [x_n_a_4] -> Sum116/1
  Mux96/1 -> Sum114/2
  Sum113/1 -> Mux96/1
  [x_n_a_3] -> Sum114/1
  [n_s1_3] -> Sum113/2
  Constant53/1 -> Mux97/2
  Mux97/1 -> Sum116/2
  [n_s1_4] -> Sum115/2
  Sum114/1 -> [f_3]
  [u_s1_7] -> Sum121/1
  Sum124/1 -> [f_8]
  [u_s1_8] -> Sum123/1
  [x_n_a_6] -> Sum120/1
  Mux98/1 -> Sum118/2
  Sum121/1 -> Mux100/1
  Sum120/1 -> [f_6]
  [x_n_a_5] -> Sum118/1
  [n_s1_5] -> Sum117/2
  Constant56/1 -> Mux100/2
  [n_s1_8] -> Sum123/2
  Sum119/1 -> Mux99/1
  [x_n_a_7] -> Sum122/1
  [u_s1_6] -> Sum119/1
  Constant57/1 -> Mux101/2
  [u_s1_5] -> Sum117/1
  [n_s1_6] -> Sum119/2
  Sum123/1 -> Mux101/1
  Sum118/1 -> [f_5]
  Mux101/1 -> Sum124/2
  Mux100/1 -> Sum122/2
  Sum117/1 -> Mux98/1
  Constant54/1 -> Mux98/2
  Constant55/1 -> Mux99/2
  Mux99/1 -> Sum120/2
  [x_n_a_8] -> Sum124/1
  Sum122/1 -> [f_7]
  [n_s1_7] -> Sum121/2
  [x_n_a_9] -> Sum126/1
  Constant59/1 -> Mux103/2
  Mux103/1 -> Sum128/2
  Sum126/1 -> [f_9]
  Sum128/1 -> [f_10]
  [x_n_a_10] -> Sum128/1
  [n_s1_10] -> Sum127/2
  Mux102/1 -> Sum126/2
  Sum125/1 -> Mux102/1
  Constant58/1 -> Mux102/2
  [u_s1_9] -> Sum125/1
  [n_s1_9] -> Sum125/2
  Sum127/1 -> Mux103/1
  [u_s1_10] -> Sum127/1
  [u_s1_5] -> Mux104/5
  [u_s1_1] -> Mux104/1
  [u_s1_4] -> Mux104/4
  [u_s1_2] -> Mux104/2
  [u_s1_7] -> Mux104/7
  [u_s1_10] -> Mux104/10
  [u_s1_3] -> Mux104/3
  [u_s1_9] -> Mux104/9
  [u_s1_8] -> Mux104/8
  [u_s1_6] -> Mux104/6
  Mux104/1 -> To Workspace2/1, MPC commands to NRF/1
  [clk] -> Mux47/4
  [clk] -> Mux49/4
  [clk] -> Mux53/4
  [clk] -> Mux58/4
  [clk] -> Mux62/4
  [clk] -> Mux66/4
  [clk] -> Mux70/4
  [clk] -> Mux74/4
  [clk] -> Mux78/4
  [clk] -> Mux82/4
  [u_s2_5] -> Mux105/5
  Mux105/1 -> To Workspace1/1, MPC commands to platoon/1
  [u_s2_7] -> Mux105/7
  [u_s2_10] -> Mux105/10
  [u_s2_2] -> Mux105/2
  [u_s2_3] -> Mux105/3
  [u_s2_9] -> Mux105/9
  [u_s2_6] -> Mux105/6
  [u_s2_1] -> Mux105/1
  [u_s2_4] -> Mux105/4
  [u_s2_8] -> Mux105/8
  [x_4] -> Gain146/1
  Gain145/1 -> Sum3/2
  [x_6] -> Gain149/1
  Gain151/1 -> Sum130/1
  Gain157/1 -> Sum137/2
  [x_3] -> Gain143/1
  Gain141/1 -> Sum7/1
  Sum3/1 -> Sum22/1
  [x_2] -> Gain158/1
  Sum7/1 -> Sum13/1
  Constant69/1 -> Sum138/2
  Gain146/1 -> Sum52/1
  Sum136/1 -> Sum54/1
  Gain154/1 -> Sum134/2
  Gain144/1 -> Sum3/1
  Gain143/1 -> Sum55/2
  Constant68/1 -> Sum135/2
  Gain139/1 -> Sum10/2
  [x_5] -> Gain148/1
  [x_7] -> Gain150/1
  [x_8] -> Gain153/1
  [x_3] -> Gain144/1
  Constant64/1 -> Sum53/2
  Sum138/1 -> Mux13/10
  Gain152/1 -> Sum130/2
  [x_10] -> Gain157/1
  Gain148/1 -> Sum131/1
  [x_6] -> Gain155/1
  Sum54/1 -> Mux13/7
  Sum129/1 -> Mux13/1
  Gain150/1 -> Sum136/2
  Sum133/1 -> Mux13/8
  [x_1] -> Gain139/1
  Constant60/1 -> Sum129/2
  Gain149/1 -> Sum131/2
  [x_9] -> Gain154/1
  Gain158/1 -> Sum55/1
  Sum22/1 -> Mux13/4
  [x_9] -> Gain156/1
  [x_1] -> Gain141/1
  Sum131/1 -> Sum132/1
  Constant66/1 -> Sum54/2
  Gain153/1 -> Sum134/1
  Sum13/1 -> Mux13/2
  Sum52/1 -> Sum53/1
  Gain156/1 -> Sum137/1
  [x_4] -> Gain145/1
  Gain142/1 -> Sum7/2
  [x_7] -> Gain151/1
  Constant63/1 -> Sum22/2
  Constant61/1 -> Sum13/2
  Sum137/1 -> Sum138/1
  Constant67/1 -> Sum133/2
  Sum134/1 -> Sum135/1
  Sum130/1 -> Sum133/1
  [x_2] -> Gain142/1
  Sum135/1 -> Mux13/9
  Gain155/1 -> Sum136/1
  Sum10/1 -> Sum129/1
  Sum53/1 -> Mux13/5
  Constant65/1 -> Sum132/2
  [r] -> Sum10/1
  Constant62/1 -> Sum2/2
  Sum55/1 -> Sum2/1
  Gain147/1 -> Sum52/2
  Mux13/1 -> headway_based_distances/1
  [x_5] -> Gain147/1
  Sum2/1 -> Mux13/3
  Sum132/1 -> Mux13/6
  [x_8] -> Gain152/1
  Gain119/1 -> Mux106/3
  Gain111/1 -> Mux106/5
  Gain116/1 -> Mux106/10
  [x_7] -> Gain113/1
  [x_6] -> Gain112/1
  [x_8] -> Gain114/1
  Gain113/1 -> Mux106/7
  Gain118/1 -> Mux106/2
  Gain114/1 -> Mux106/8
  Gain120/1 -> Mux106/4
  Gain115/1 -> Mux106/9
  Mux106/1 -> To Workspace4/1, vehicle speed/1
  [x_9] -> Gain115/1
  [x_5] -> Gain111/1
  [x_10] -> Gain116/1
  [x_3] -> Gain119/1
  [x_1] -> Gain117/1
  Gain117/1 -> Mux106/1
  Gain112/1 -> Mux106/6
  [x_2] -> Gain118/1
  [x_4] -> Gain120/1
  Fcn/1 -> Gain17/1, Discrete-Time Integrator1/1
  Clock1/1 -> Fcn/1, [clk]
  Discrete-Time Integrator1/1 -> [r]
  Gain17/1 -> [d_r]
  [x_6] -> Gain45/1
  Sum157/1 -> Sum151/1
  Sum145/1 -> Mux107/8
  Gain20/1 -> Sum158/2
  [x_10] -> Gain47/1
  [r] -> Sum139/1
  Sum158/1 -> Sum141/1
  Gain46/1 -> Sum149/1
  Gain19/1 -> Sum158/1
  Constant77/1 -> Sum145/2
  Gain24/1 -> Sum154/1
  Constant75/1 -> Sum144/2
  Sum154/1 -> Sum155/1
  Constant74/1 -> Sum155/2
  Sum139/1 -> Sum140/1
  Gain43/1 -> Sum146/1
  Gain26/1 -> Sum143/1
  Sum148/1 -> Sum156/1
  Gain22/1 -> Sum153/1
  Constant71/1 -> Sum141/2
  [x_5] -> Gain25/1
  [x_8] -> Gain43/1
  Sum147/1 -> Mux107/9
  [x_8] -> Gain42/1
  Gain71/1 -> Sum157/1
  [x_5] -> Gain26/1
  Gain27/1 -> Sum143/2
  Gain21/1 -> Sum157/2
  [x_6] -> Gain27/1
  Sum142/1 -> Sum145/1
  Constant72/1 -> Sum151/2
  [x_9] -> Gain46/1
  Gain42/1 -> Sum142/2
  Gain25/1 -> Sum154/2
  Constant78/1 -> Sum147/2
  [x_7] -> Gain39/1
  [x_1] -> Gain18/1
  Sum140/1 -> Mux107/1
  Gain44/1 -> Sum146/2
  Constant79/1 -> Sum150/2
  Sum149/1 -> Sum150/1
  Sum151/1 -> Mux107/3
  Gain23/1 -> Sum153/2
  [x_3] -> Gain22/1
  [x_4] -> Gain23/1
  Mux107/1 -> To Workspace/1, length_based_interdistances/1
  Sum146/1 -> Sum147/1
  Gain18/1 -> Sum139/2
  Constant70/1 -> Sum140/2
  Gain45/1 -> Sum148/1
  Sum152/1 -> Mux107/4
  [x_2] -> Gain71/1
  Constant76/1 -> Sum156/2
  [x_3] -> Gain21/1
  Constant73/1 -> Sum152/2
  Gain38/1 -> Sum148/2
  Gain47/1 -> Sum149/2
  Sum155/1 -> Mux107/5
  Sum143/1 -> Sum144/1
  [x_4] -> Gain24/1
  Sum156/1 -> Mux107/7
  Sum141/1 -> Mux107/2
  Sum153/1 -> Sum152/1
  Sum150/1 -> Mux107/10
  Sum144/1 -> Mux107/6
  [x_1] -> Gain19/1
  Gain39/1 -> Sum142/1
  [x_2] -> Gain20/1
  [x_7] -> Gain38/1
  [x_9] -> Gain44/1
